simulink model "Populationsmodell"  (R2024b)
settings: Solver=VariableStepAuto  StartTime=0.0  StopTime=100  RelTol=1e-3
settings Model: Creator=marvincalmer  LastModifiedBy=marvincalmer

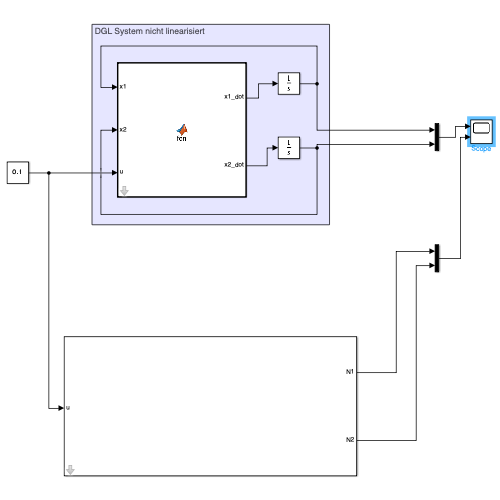
[thumbnail: Simulink's stored preview of the top-level diagram]
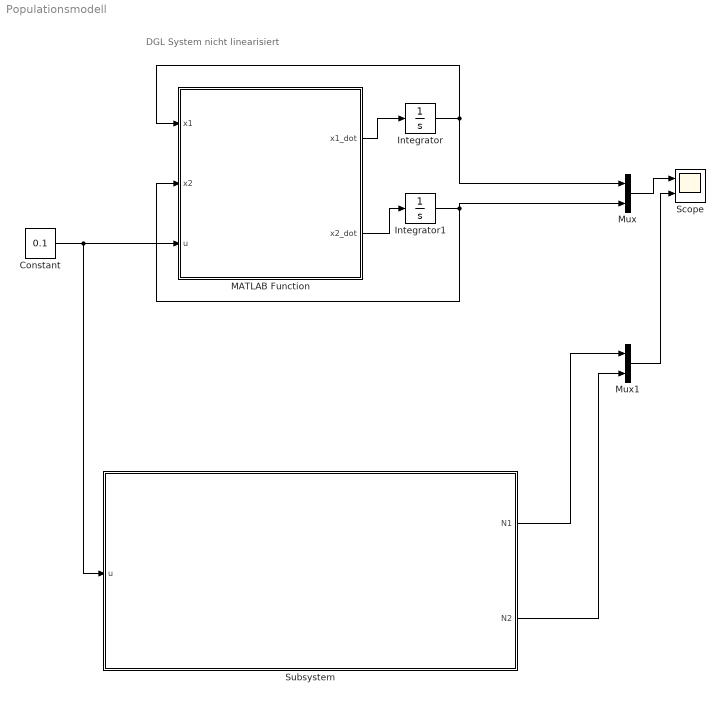
== system Populationsmodell ==
  note: DGL System nicht linearisiert
  Constant : Constant  Value=0.1
  Integrator : Integrator  InitialCondition=40
  Integrator1 : Integrator  InitialCondition=9
  MATLAB Function : MATLAB Function  TreatAsAtomicUnit=on  mask{x10=10, x20=10, epsilon1=1, epsilon2=0.5, gamm1=0.05, gamm2=0.02, e=0.2, f=0.1}
      mask prompts: x10 "Startwert 1"; x20 "Startwert 2"; gamm1 "gamma1"; gamm2 "gamma2"
  Mux : Mux  Inputs=2
  Mux1 : Mux  Inputs=2
  Scope : Scope  NumInputPorts=2
  Subsystem : Subsystem  mask{e=0.2, f=0.1, gamm1=0.05, gamm2=0.02, epsilon1=1, epsilon2=0.5}
      mask prompts: gamm1 "gamma1"; gamm2 "gamma2"; epsilon2 "epsilon1"
  wires:
  MATLAB Function/2(x2_dot) -> Integrator1/1
  Integrator1/1 -> MATLAB Function/2(x2), Mux/2
  Constant/1 -> Subsystem/1(u), MATLAB Function/3(u)
  MATLAB Function/1(x1_dot) -> Integrator/1
  Integrator/1 -> Mux/1, MATLAB Function/1(x1)
  Mux/1 -> Scope/1
  Subsystem/1(N1) -> Mux1/1
  Subsystem/2(N2) -> Mux1/2
  Mux1/1 -> Scope/2

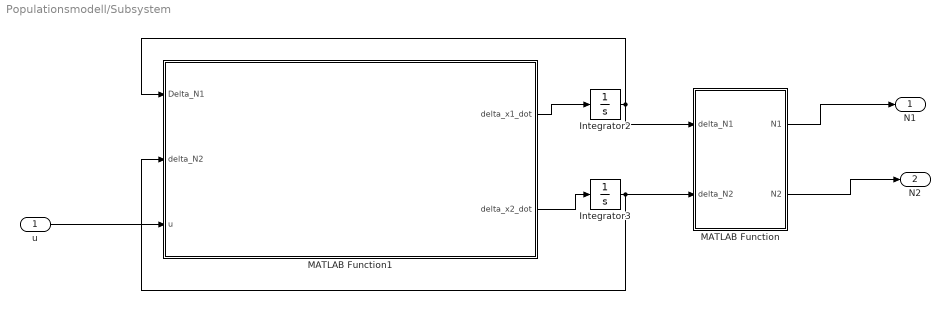
== system Populationsmodell/Subsystem ==
  u : Inport
  Integrator2 : Integrator  InitialCondition=40
  Integrator3 : Integrator  InitialCondition=9
  MATLAB Function : MATLAB Function  TreatAsAtomicUnit=on
  MATLAB Function1 : MATLAB Function  TreatAsAtomicUnit=on
  N1 : Outport
  N2 : Outport  Port=2
  wires:
  Integrator2/1 -> MATLAB Function1/1(Delta_N1), MATLAB Function/1(delta_N1)
  MATLAB Function1/1(delta_x1_dot) -> Integrator2/1
  MATLAB Function1/2(delta_x2_dot) -> Integrator3/1
  Integrator3/1 -> MATLAB Function1/2(delta_N2), MATLAB Function/2(delta_N2)
  u/1 -> MATLAB Function1/3(u)
  MATLAB Function/1(N1) -> N1/1
  MATLAB Function/2(N2) -> N2/1

== matlab function Populationsmodell/Subsystem/MATLAB Function ==
  data: delta_N1 input; N1 output; delta_N2 input; N2 output; epsilon1 parameter; epsilon2 parameter; gamm1 parameter; gamm2 parameter
function [N1,N2] = fcn(delta_N1,delta_N2,epsilon1, epsilon2, gamm1, gamm2)
    N1=delta_N1+epsilon2/gamm2;
    N2=delta_N2+epsilon1/gamm1;
end

== matlab function Populationsmodell/MATLAB Function ==
  data: x1 input; x2 input; u input; x1_dot output; x2_dot output; epsilon1 parameter; epsilon2 parameter; gamm1 parameter; gamm2 parameter; e parameter; f parameter
function [x1_dot,x2_dot] = fcn(x1,x2,u,epsilon1, epsilon2, gamm1, gamm2, e, f)

x1_dot=epsilon1*x1-gamm1*x1*x2-e*u;
x2_dot=gamm2*x1*x2-epsilon2*x2-f*u;


end

== matlab function Populationsmodell/Subsystem/MATLAB Function1 ==
  data: Delta_N1 input; delta_N2 input; u input; delta_x1_dot output; delta_x2_dot output; epsilon1 parameter; epsilon2 parameter; gamm1 parameter; gamm2 parameter; e parameter; f parameter
function [delta_x1_dot,delta_x2_dot] = fcn(Delta_N1,delta_N2,u,epsilon1, epsilon2, gamm1, gamm2, e, f)

us = 0;
delta_us=u-us;

a11 = 0;
a12 = -epsilon2*gamm1/gamm2;
a21 = gamm2*epsilon1/gamm1;
a22 = 0;

b1=-e;
b2=-f;

delta_x1_dot=a11*Delta_N1 + a12*delta_N2+delta_us*b1;
delta_x2_dot=a21*Delta_N1 + a22*delta_N2+delta_us*b2;


end
